simulink model "NL_After_OHC_Function"  (R2019b)
settings: Solver=VariableStepAuto  StartTime=0.0  StopTime=testtime  RelTol=1e-3
InitFcn:
  | NL_After_OHC_Test_Parameters
StopFcn:
  | Verify_NL_After_OHC_Function
values from neighbouring files (symbols this model uses):
  Fs = 48e3    (= 48000)    [NL_After_OHC_Test_Parameters.m]
  minR = 0.05    [NL_After_OHC_Test_Parameters.m]
  minRout = halfR    [NL_After_OHC_Test_Parameters.m]
  ohcasym = 7.0    (= 7)    [NL_After_OHC_Test_Parameters.m]
  R = taumin./taumax    [NL_After_OHC_Test_Parameters.m]
  taumax = 0.003    [NL_After_OHC_Test_Parameters.m]
  taumin = 4.6310e-04    (= 0.0004631)    [NL_After_OHC_Test_Parameters.m]
libraries: dspsrcs4 x2
settings Model: Creator=mblun  LastModifiedBy=The Awesome One
settings OptimizationCC: BlockReduction=off  ConditionallyExecuteInputs=off  DefaultParameterBehavior=Inlined
settings DebuggingCC: AlgebraicLoopMsg=error
settings HardwareCC: ProdBitPerPointer=32  ProdBitPerSizeT=32  ProdBitPerPtrDiffT=32  ProdLargestAtomicFloat=None  ProdIntDivRoundTo=Undefined  ProdEndianess=Unspecified  ProdWordSize=32  ProdHWDeviceType=ASIC/FPGA->ASIC/FPGA  TargetBitPerPointer=64  TargetBitPerSizeT=64  TargetBitPerPtrDiffT=64  TargetLongLongMode=on  TargetIntDivRoundTo=Zero  TargetEndianess=LittleEndian  TargetWordSize=64  TargetHWDeviceType=Custom Processor->MATLAB Host Computer  ProdEqTarget=off
settings SFSimCC: CustomCodeUndefinedFunction=UseInterfaceOnly

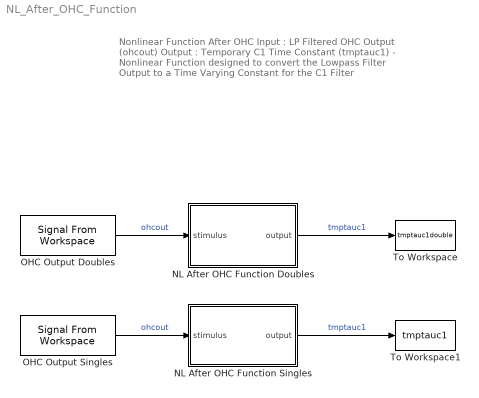
== system NL_After_OHC_Function ==
  note: Nonlinear Function After OHC
      |
      | Input : LP Filtered OHC Output (ohcout)
      |
      | Output : Temporary C1 Time Constant (tmptauc1)
      |
      | - Nonlinear Function designed to convert the Lowpass Filter Output to a Time Varying Constant for the C1 Filter
  NL After OHC Function Doubles : Subsystem
  NL After OHC Function Singles : Subsystem
  OHC Output Doubles : dspsrcs4/Signal From Workspace  X=RxSignalDouble  Ts=1/Fs  nsamps=1  OutputAfterFinalValue=Setting to zero  ignoreOrWarnInputAndFrameLengths=off  OutputFrames=off
  OHC Output Singles : dspsrcs4/Signal From Workspace  X=RxSignal  Ts=1/Fs  nsamps=1  OutputAfterFinalValue=Setting to zero  ignoreOrWarnInputAndFrameLengths=off  OutputFrames=off
  To Workspace : ToWorkspace  VariableName=tmptauc1double  SampleTime=-1
      settings: Save2DSignal=2-D array (concatenate along first dimension)
  To Workspace1 : ToWorkspace  VariableName=tmptauc1  SampleTime=-1
      settings: Save2DSignal=2-D array (concatenate along first dimension)
  wires:
  OHC Output Doubles/1 -> NL After OHC Function Doubles/1(stimulus)  "ohcout"
  NL After OHC Function Doubles/1(output) -> To Workspace/1  "tmptauc1"
  OHC Output Singles/1 -> NL After OHC Function Singles/1(stimulus)  "ohcout"
  NL After OHC Function Singles/1(output) -> To Workspace1/1  "tmptauc1"

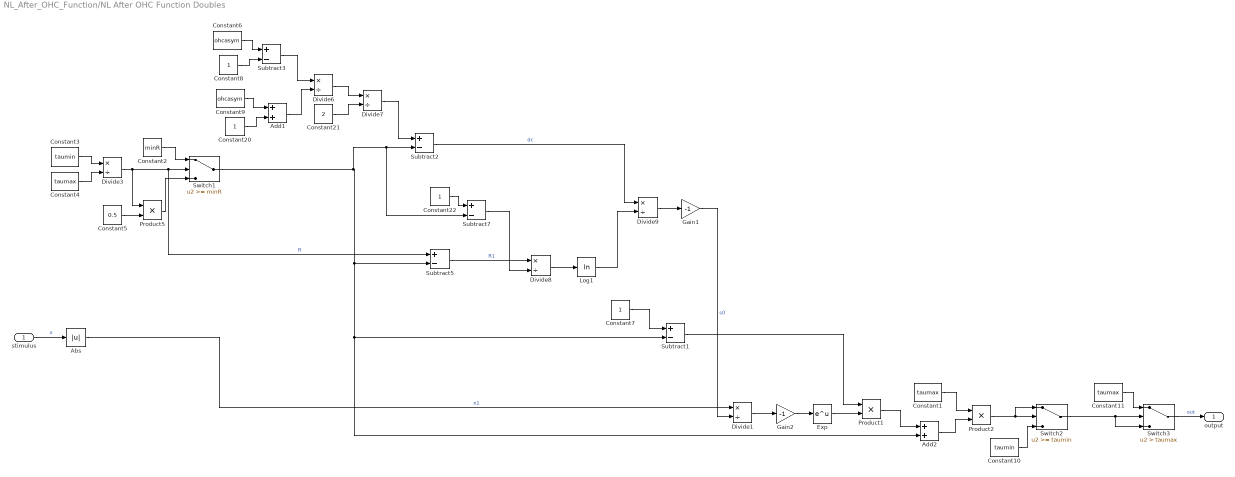
== system NL_After_OHC_Function/NL After OHC Function Doubles ==
  stimulus : Inport
  Abs : Abs
  Add1 : Sum
  Add2 : Sum
  Constant1 : Constant  Value=taumax  SampleTime=-1
  Constant10 : Constant  Value=taumin  SampleTime=-1
  Constant11 : Constant  Value=taumax  SampleTime=-1
  Constant2 : Constant  Value=minR  SampleTime=-1
  Constant{7..8,20,22} (4 alike) : Constant  SampleTime=-1
  Constant21 : Constant  Value=2  SampleTime=-1
  Constant3 : Constant  Value=taumin  SampleTime=-1
  Constant4 : Constant  Value=taumax  SampleTime=-1
  Constant5 : Constant  Value=0.5  SampleTime=-1
  Constant6 : Constant  Value=ohcasym  SampleTime=-1
  Constant9 : Constant  Value=ohcasym  SampleTime=-1
  Divide{1,3,6..9} (6 alike) : Product  Inputs=*/  SaturateOnIntegerOverflow=on  RndMeth=Zero
  Exp : Math  SaturateOnIntegerOverflow=on
  Gain1 : Gain  Gain=-1
  Gain2 : Gain  Gain=-1
  Log1 : Math  Operator=log  SaturateOnIntegerOverflow=on
  Product1 : Product
  Product2 : Product
  Product5 : Product
  Subtract{1..3,5,7} (5 alike) : Sum  Inputs=+-
  Switch1 : Switch  Threshold=minR
  Switch2 : Switch  Threshold=taumin
  Switch3 : Switch  Criteria=u2 > Threshold  Threshold=taumax
  output : Outport  VectorParamsAs1DForOutWhenUnconnected=off
  wires:
  Constant3/1 -> Divide3/1
  Constant4/1 -> Divide3/2
  Divide3/1 -> Subtract5/1, Switch1/2, Product5/1  "R"
  Constant2/1 -> Switch1/1
  Constant5/1 -> Product5/2
  Product5/1 -> Switch1/3
  Switch1/1 -> Subtract7/2, Subtract2/2, Add2/2, Subtract1/2, Subtract5/2
  Constant8/1 -> Subtract3/2
  Constant6/1 -> Subtract3/1
  Constant20/1 -> Add1/2
  Constant9/1 -> Add1/1
  Subtract3/1 -> Divide6/1
  Add1/1 -> Divide6/2
  Divide6/1 -> Divide7/1
  Constant21/1 -> Divide7/2
  Divide7/1 -> Subtract2/1
  Subtract2/1 -> Divide9/1  "dc"
  Subtract5/1 -> Divide8/1  "R1"
  Constant22/1 -> Subtract7/1
  Subtract7/1 -> Divide8/2
  Divide8/1 -> Log1/1
  Log1/1 -> Divide9/2
  Divide9/1 -> Gain1/1
  Gain1/1 -> Divide1/2  "s0"
  stimulus/1 -> Abs/1  "x"
  Abs/1 -> Divide1/1  "x1"
  Constant7/1 -> Subtract1/1
  Divide1/1 -> Gain2/1
  Gain2/1 -> Exp/1
  Subtract1/1 -> Product1/1
  Exp/1 -> Product1/2
  Product1/1 -> Add2/1
  Constant1/1 -> Product2/1
  Add2/1 -> Product2/2
  Product2/1 -> Switch2/1, Switch2/2
  Constant10/1 -> Switch2/3
  Switch2/1 -> Switch3/3, Switch3/2
  Constant11/1 -> Switch3/1
  Switch3/1 -> output/1  "out"

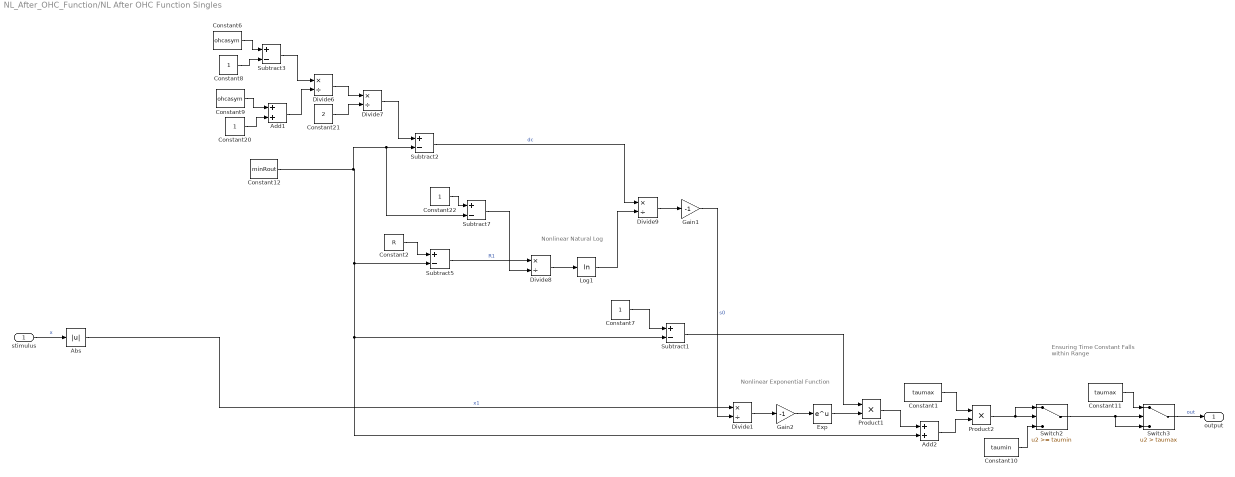
== system NL_After_OHC_Function/NL After OHC Function Singles ==
  note: Ensuring Time Constant Falls within Range
  note: Nonlinear Natural Log
  note: Nonlinear Exponential Function
  stimulus : Inport
  Abs : Abs
  Add1 : Sum
  Add2 : Sum
  Constant1 : Constant  Value=taumax  OutDataTypeStr=single  SampleTime=-1
  Constant10 : Constant  Value=taumin  OutDataTypeStr=single  SampleTime=-1
  Constant11 : Constant  Value=taumax  OutDataTypeStr=single  SampleTime=-1
  Constant12 : Constant  Value=minRout  OutDataTypeStr=single  SampleTime=-1
  Constant2 : Constant  Value=R  OutDataTypeStr=single  SampleTime=-1
  Constant{7..8,20,22} (4 alike) : Constant  OutDataTypeStr=single  SampleTime=-1
  Constant21 : Constant  Value=2  OutDataTypeStr=single  SampleTime=-1
  Constant6 : Constant  Value=ohcasym  OutDataTypeStr=single  SampleTime=-1
  Constant9 : Constant  Value=ohcasym  OutDataTypeStr=single  SampleTime=-1
  Divide{1,6..9} (5 alike) : Product  Inputs=*/  SaturateOnIntegerOverflow=on  RndMeth=Zero
  Exp : Math  SaturateOnIntegerOverflow=on
  Gain1 : Gain  Gain=-1
  Gain2 : Gain  Gain=-1
  Log1 : Math  Operator=log  SaturateOnIntegerOverflow=on
  Product1 : Product
  Product2 : Product
  Subtract{1..3,5,7} (5 alike) : Sum  Inputs=+-
  Switch2 : Switch  Threshold=taumin
  Switch3 : Switch  Criteria=u2 > Threshold  Threshold=taumax
  output : Outport  VectorParamsAs1DForOutWhenUnconnected=off
  wires:
  Constant12/1 -> Subtract7/2, Subtract2/2, Add2/2, Subtract1/2, Subtract5/2
  Constant8/1 -> Subtract3/2
  Constant6/1 -> Subtract3/1
  Constant20/1 -> Add1/2
  Constant9/1 -> Add1/1
  Subtract3/1 -> Divide6/1
  Add1/1 -> Divide6/2
  Divide6/1 -> Divide7/1
  Constant21/1 -> Divide7/2
  Divide7/1 -> Subtract2/1
  Subtract2/1 -> Divide9/1  "dc"
  Subtract5/1 -> Divide8/1  "R1"
  Constant22/1 -> Subtract7/1
  Subtract7/1 -> Divide8/2
  Divide8/1 -> Log1/1
  Log1/1 -> Divide9/2
  Divide9/1 -> Gain1/1
  Gain1/1 -> Divide1/2  "s0"
  stimulus/1 -> Abs/1  "x"
  Abs/1 -> Divide1/1  "x1"
  Constant7/1 -> Subtract1/1
  Divide1/1 -> Gain2/1
  Gain2/1 -> Exp/1
  Subtract1/1 -> Product1/1
  Exp/1 -> Product1/2
  Product1/1 -> Add2/1
  Constant1/1 -> Product2/1
  Add2/1 -> Product2/2
  Product2/1 -> Switch2/1, Switch2/2
  Constant10/1 -> Switch2/3
  Switch2/1 -> Switch3/3, Switch3/2
  Constant11/1 -> Switch3/1
  Switch3/1 -> output/1  "out"
  Constant2/1 -> Subtract5/1
